simulink library "MOVH"  (R2016b)
settings: Solver=ode45  StartTime=0.0  StopTime=10.0  RelTol=1e-3  EnableMultiTasking=on
undefined symbols (not defined in the file): CAL_fullCircle_DEG, CAL_halfCircle_DEG, CAL_Kd, CAL_Ki, CAL_Kp, CAL_NO_ERROR, CAL_thetaGain, CONST_EnableDelay, CONST_NegOne, CONST_TWO_F32, CONST_ZERO_F32, ENU_BACKWARD, ENU_CCW, ENU_CW, ENU_FORWARD, ENU_MOVE_TURN_LEFT, ENU_MOVE_TURN_RIGHT, ENU_MOVE_U_TURN, ENU_MOVE_U_TURN_LEFT, ENU_MOVE_U_TURN_RIGHT, ENU_ROB_NONE, ENU_STOP
libraries: simulink_need_slupdate x2
settings Model: Creator=oelkawok  LastModifiedBy=oelkawok
settings DataIOCC: LimitDataPoints=on
settings OptimizationCC: LifeSpan=inf
settings DebuggingCC: AllowSymbolicDim=off  SFUnexpectedBacktrackingDiag=warning  SFNoUnconditionalDefaultTransitionDiag=warning  SFExecutionAtInitializationDiag=none
settings GRTTargetCC: TargetLangStandard=C89/C90 (ANSI)  GeneratePreprocessorConditionals=Disable all
settings ConfigComp: CovMetricSettings=dw  CovHtmlReporting=on  CovSaveCumulativeToWorkspaceVar=on  CovSaveSingleToWorkspaceVar=on  CovExternalEMLEnable=off

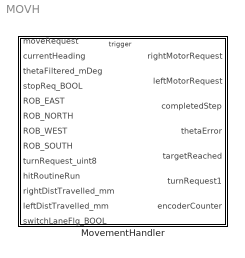
== system MOVH ==
  MovementHandler : Subsystem

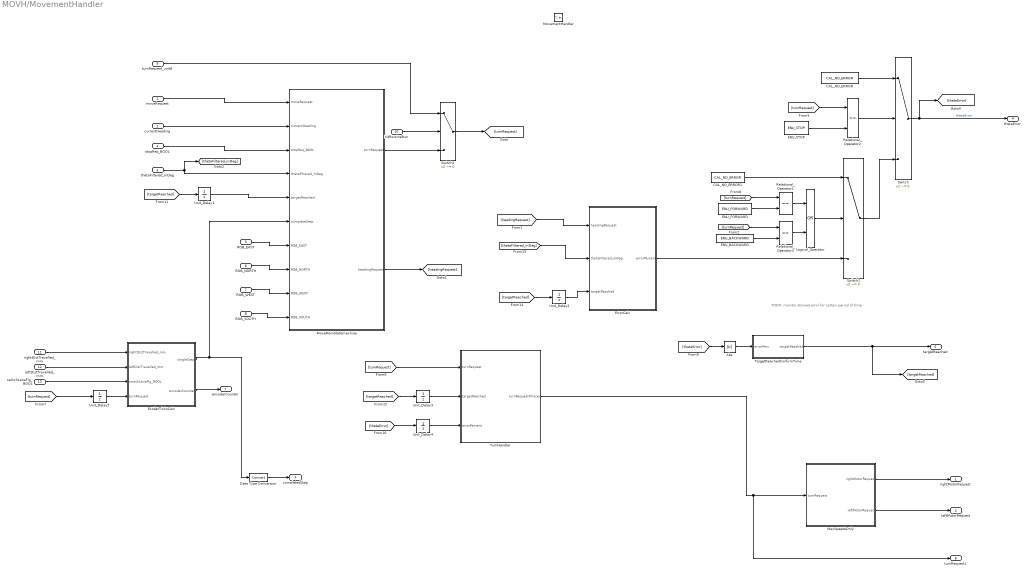
== system MOVH/MovementHandler ==
  note: TODO: monitor allowed error for certain period of time
  moveRequest : Inport
  currentHeading : Inport  Port=2
  thetaFiltered_mDeg : Inport  Port=3  PortDimensions=1
  stopReq_BOOL : Inport  Port=4
  ROB_EAST : Inport  Port=5  PortDimensions=1
  ROB_NORTH : Inport  Port=6  PortDimensions=1
  ROB_WEST : Inport  Port=7  PortDimensions=1
  ROB_SOUTH : Inport  Port=8  PortDimensions=1
  turnRequest_uint8 : Inport  Port=9
  hitRoutineRun : Inport  Port=10
  rightDistTravelled_mm : Inport  Port=11  PortDimensions=1
  leftDistTravelled_mm : Inport  Port=12  PortDimensions=1
  switchLaneFlg_BOOL : Inport  Port=13  PortDimensions=1
  MovementHandler : TriggerPort  TriggerType=function-call  VariantControl=Variant
      settings: AttributesFormatString=Mode: %<StatesWhenEnabling>
  Abs : Abs
  CAL_NO_ERROR : Constant  Value=CAL_NO_ERROR
  CAL_NO_ERROR1 : Constant  Value=CAL_NO_ERROR
  Data Type Conversion : DataTypeConversion
  ENU_BACKWARD : Constant  Value=ENU_BACKWARD
  ENU_FORWARD : Constant  Value=ENU_FORWARD
  ENU_STOP : Constant  Value=ENU_STOP
  EcoderTicksCalc : Subsystem
  ErrorCalc : Subsystem
  Logical_Operator : Logic  Operator=OR  AllPortsSameDT=off  OutDataTypeStr=boolean
  MaxSpeedsOnly : Subsystem
  MoveMainStatemachine : Subsystem
  Relational_Operator1 : RelationalOperator  Operator===  OutDataTypeStr=boolean  RndMeth=Nearest
  Relational_Operator2 : RelationalOperator  Operator===  OutDataTypeStr=boolean  RndMeth=Nearest
  Relational_Operator3 : RelationalOperator  Operator===  OutDataTypeStr=boolean  RndMeth=Nearest
  Switch : Switch  Criteria=u2 ~= 0
  Switch1 : Switch  Criteria=u2 ~= 0
  Switch2 : Switch  Criteria=u2 ~= 0
  TargetReachedConfirmTime : Subsystem
  TurnHandler : Subsystem
  Unit_Delay{1..4} (4 alike) : UnitDelay  InitialCondition=CAL_NO_ERROR  SampleTime=-1
      settings: AttributesFormatString=Init: %<InitialCondition>
  Unit_Delay5 : UnitDelay  InitialCondition=false  SampleTime=-1
      settings: AttributesFormatString=Init: %<InitialCondition>
  rightMotorRequest : Outport
      settings: AttributesFormatString=|
      | Mode: %<OutputWhenDisabled>
      | Init: %<InitialOutput>
  leftMotorRequest : Outport  Port=2
      settings: AttributesFormatString=|
      | Mode: %<OutputWhenDisabled>
      | Init: %<InitialOutput>
  completedStep : Outport  Port=3
      settings: AttributesFormatString=|
      | Mode: %<OutputWhenDisabled>
      | Init: %<InitialOutput>
  thetaError : Outport  Port=4  OutputWhenDisabled=reset  InitialOutput=0
      settings: AttributesFormatString=|
      | Mode: %<OutputWhenDisabled>
      | Init: %<InitialOutput>
  targetReached : Outport  Port=5  OutputWhenDisabled=reset  InitialOutput=0
      settings: AttributesFormatString=|
      | Mode: %<OutputWhenDisabled>
      | Init: %<InitialOutput>
  turnRequest1 : Outport  Port=6
      settings: AttributesFormatString=|
      | Mode: %<OutputWhenDisabled>
      | Init: %<InitialOutput>
  encoderCounter : Outport  Port=7
      settings: AttributesFormatString=|
      | Mode: %<OutputWhenDisabled>
      | Init: %<InitialOutput>
  wires:
  Logical_Operator/1 -> Switch1/2
  Abs/1 -> TargetReachedConfirmTime/1(errorPerc)
  TargetReachedConfirmTime/1(targetReached) -> targetReached/1, [targetReached]
  Data Type Conversion/1 -> completedStep/1
  Unit_Delay1/1 -> MoveMainStatemachine/5(targetReached)
  [targetReached] -> Unit_Delay1/1
  [thetaFiltered_mDeg] -> ErrorCalc/2(thetaFiltered_mDeg)
  thetaFiltered_mDeg/1 -> [thetaFiltered_mDeg], MoveMainStatemachine/4(thetaFiltered_mDeg)
  currentHeading/1 -> MoveMainStatemachine/2(currentHeading)
  MoveMainStatemachine/2(headingRequest) -> [headingRequest]
  MoveMainStatemachine/1(turnRequest) -> Switch2/3
  stopReq_BOOL/1 -> MoveMainStatemachine/3(stopReq_BOOL)
  moveRequest/1 -> MoveMainStatemachine/1(moveRequest)
  MaxSpeedsOnly/1(rightMotorRequest) -> rightMotorRequest/1
  MaxSpeedsOnly/2(leftMotorRequest) -> leftMotorRequest/1
  [turnRequest] -> TurnHandler/1(turnRequest)
  [headingRequest] -> ErrorCalc/1(headingRequest)
  ENU_STOP/1 -> Relational_Operator2/2
  [turnRequest] -> Relational_Operator2/1
  Relational_Operator2/1 -> Switch/2
  CAL_NO_ERROR/1 -> Switch/1
  Switch1/1 -> Switch/3
  [turnRequest] -> Relational_Operator1/1
  ErrorCalc/1(errorPercent) -> Switch1/3
  Switch/1 -> [thetaError], thetaError/1  "thetaError"
  [thetaError] -> Abs/1
  [targetReached] -> Unit_Delay2/1
  Unit_Delay2/1 -> ErrorCalc/3(targetReached)
  [targetReached] -> Unit_Delay3/1
  Unit_Delay3/1 -> TurnHandler/2(targetReached)
  Unit_Delay4/1 -> TurnHandler/3(errorPercent)
  [thetaError] -> Unit_Delay4/1
  TurnHandler/1(turnRequestFiltered) -> MaxSpeedsOnly/1(turnRequest), turnRequest1/1
  CAL_NO_ERROR1/1 -> Switch1/1
  EcoderTicksCalc/1(singleStep) -> Data Type Conversion/1, MoveMainStatemachine/6(completeStep)
  ROB_EAST/1 -> MoveMainStatemachine/7(ROB_EAST)
  ROB_NORTH/1 -> MoveMainStatemachine/8(ROB_NORTH)
  ROB_WEST/1 -> MoveMainStatemachine/9(ROB_WEST)
  ROB_SOUTH/1 -> MoveMainStatemachine/10(ROB_SOUTH)
  turnRequest_uint8/1 -> Switch2/1
  Switch2/1 -> [turnRequest]
  hitRoutineRun/1 -> Switch2/2
  EcoderTicksCalc/2(encoderCounter) -> encoderCounter/1
  [turnRequest] -> Unit_Delay5/1
  ENU_FORWARD/1 -> Relational_Operator1/2
  ENU_BACKWARD/1 -> Relational_Operator3/2
  [turnRequest] -> Relational_Operator3/1
  Relational_Operator1/1 -> Logical_Operator/1
  Relational_Operator3/1 -> Logical_Operator/2
  Unit_Delay5/1 -> EcoderTicksCalc/4(turnRequest)
  rightDistTravelled_mm/1 -> EcoderTicksCalc/1(rightDistTravelled_mm)
  leftDistTravelled_mm/1 -> EcoderTicksCalc/2(leftDistTravelled_mm)
  switchLaneFlg_BOOL/1 -> EcoderTicksCalc/3(switchLaneFlg_BOOL)

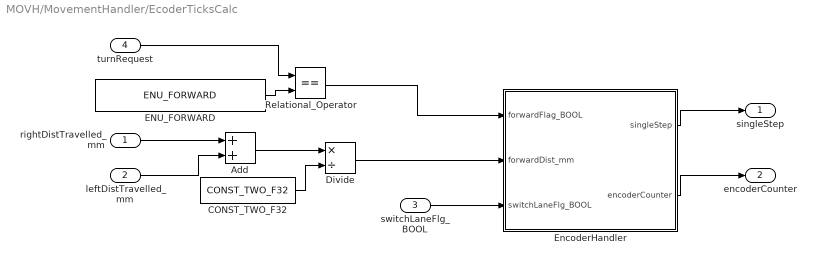
== system MOVH/MovementHandler/EcoderTicksCalc ==
  rightDistTravelled_mm : Inport  PortDimensions=1
  leftDistTravelled_mm : Inport  Port=2  PortDimensions=1
  switchLaneFlg_BOOL : Inport  Port=3  PortDimensions=1
  turnRequest : Inport  Port=4  PortDimensions=1
  Add : Sum
  CONST_TWO_F32 : Constant  Value=CONST_TWO_F32
  Divide : Product  Inputs=*/
  ENU_FORWARD : Constant  Value=ENU_FORWARD
  EncoderHandler : Subsystem
  Relational_Operator : RelationalOperator  Operator===  OutDataTypeStr=boolean  RndMeth=Simplest
  singleStep : Outport
  encoderCounter : Outport  Port=2
  wires:
  EncoderHandler/1(singleStep) -> singleStep/1
  EncoderHandler/2(encoderCounter) -> encoderCounter/1
  turnRequest/1 -> Relational_Operator/1
  rightDistTravelled_mm/1 -> Add/1
  leftDistTravelled_mm/1 -> Add/2
  Add/1 -> Divide/1
  CONST_TWO_F32/1 -> Divide/2
  ENU_FORWARD/1 -> Relational_Operator/2
  Divide/1 -> EncoderHandler/2(forwardDist_mm)
  switchLaneFlg_BOOL/1 -> EncoderHandler/3(switchLaneFlg_BOOL)
  Relational_Operator/1 -> EncoderHandler/1(forwardFlag_BOOL)

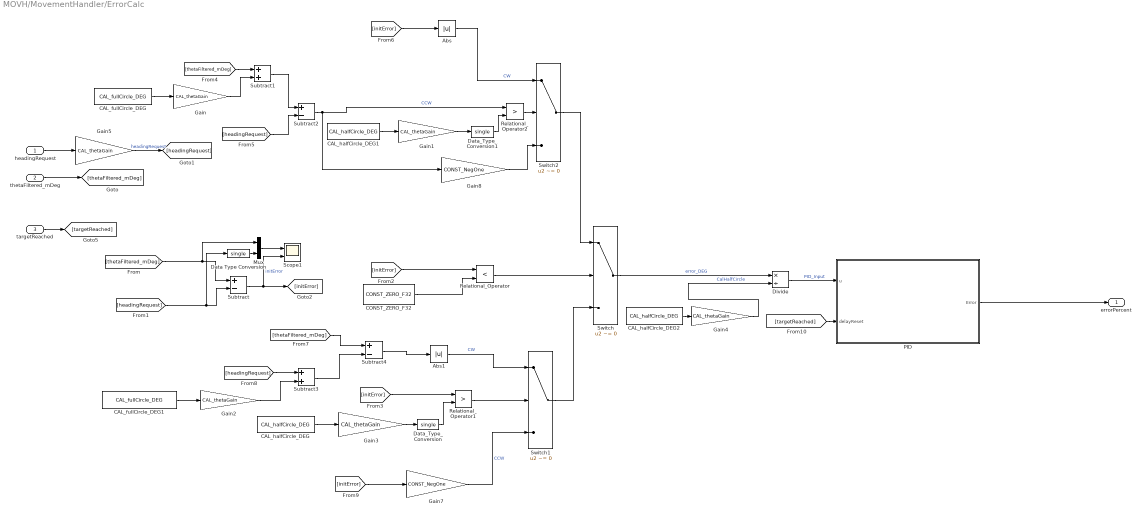
== system MOVH/MovementHandler/ErrorCalc ==
  headingRequest : Inport
  thetaFiltered_mDeg : Inport  Port=2
  targetReached : Inport  Port=3
  Abs : Abs
  Abs1 : Abs
  CAL_fullCircle_DEG : Constant  Value=CAL_fullCircle_DEG
  CAL_fullCircle_DEG1 : Constant  Value=CAL_fullCircle_DEG
  CAL_halfCircle_DEG : Constant  Value=CAL_halfCircle_DEG
  CAL_halfCircle_DEG1 : Constant  Value=CAL_halfCircle_DEG
  CAL_halfCircle_DEG2 : Constant  Value=CAL_halfCircle_DEG
  CONST_ZERO_F32 : Constant  Value=CONST_ZERO_F32
  Data Type Conversion : DataTypeConversion  OutDataTypeStr=single
  Data_Type_Conversion : DataTypeConversion  OutDataTypeStr=single
  Data_Type_Conversion1 : DataTypeConversion  OutDataTypeStr=single
  Divide : Product  Inputs=*/
  Gain : Gain  Gain=CAL_thetaGain  OutDataTypeStr=int32
  Gain1 : Gain  Gain=CAL_thetaGain  OutDataTypeStr=int16
  Gain2 : Gain  Gain=CAL_thetaGain  OutDataTypeStr=int32
  Gain3 : Gain  Gain=CAL_thetaGain  OutDataTypeStr=Inherit: Inherit via back propagation
  Gain4 : Gain  Gain=CAL_thetaGain  OutDataTypeStr=int16
  Gain5 : Gain  Gain=CAL_thetaGain  OutDataTypeStr=int32
  Gain7 : Gain  Gain=CONST_NegOne
  Gain8 : Gain  Gain=CONST_NegOne
  Mux : Mux  Inputs=2
  PID : Subsystem
  Relational_Operator : RelationalOperator  Operator=<  OutDataTypeStr=boolean  RndMeth=Nearest
  Relational_Operator1 : RelationalOperator  Operator=>  OutDataTypeStr=boolean  RndMeth=Nearest
  Relational_Operator2 : RelationalOperator  Operator=>  OutDataTypeStr=boolean  RndMeth=Nearest
  Scope1 : Scope  NumInputPorts=2
  Subtract : Sum  Inputs=+-
  Subtract1 : Sum
  Subtract2 : Sum  Inputs=+-
  Subtract3 : Sum  OutDataTypeStr=int32
  Subtract4 : Sum  Inputs=+-
  Switch : Switch  Criteria=u2 ~= 0
  Switch1 : Switch  Criteria=u2 ~= 0
  Switch2 : Switch  Criteria=u2 ~= 0
  errorPercent : Outport  OutputWhenDisabled=reset  InitialOutput=0
  wires:
  Data Type Conversion/1 -> Mux/2
  Mux/1 -> Scope1/1
  CAL_halfCircle_DEG2/1 -> Gain4/1
  Switch/1 -> Divide/1  "error_DEG"
  [initError] -> Gain7/1
  Abs1/1 -> Switch1/1  "CW"
  Subtract4/1 -> Abs1/1
  Subtract3/1 -> Subtract4/2
  [thetaFiltered_mDeg] -> Subtract4/1
  [headingRequest] -> Subtract3/1
  CAL_fullCircle_DEG1/1 -> Gain2/1
  Abs/1 -> Switch2/1  "CW"
  [initError] -> Abs/1
  Switch2/1 -> Switch/1
  Relational_Operator2/1 -> Switch2/2
  Subtract2/1 -> Relational_Operator2/1, Gain8/1  "CCW"
  CAL_halfCircle_DEG1/1 -> Gain1/1
  [headingRequest] -> Subtract2/2
  Subtract1/1 -> Subtract2/1
  CAL_fullCircle_DEG/1 -> Gain/1
  [thetaFiltered_mDeg] -> Subtract1/1
  [initError] -> Relational_Operator1/1
  [initError] -> Relational_Operator/1
  Subtract/1 -> [initError], Scope1/2  "initError"
  [thetaFiltered_mDeg] -> Subtract/1, Mux/1
  [headingRequest] -> Subtract/2, Data Type Conversion/1
  thetaFiltered_mDeg/1 -> [thetaFiltered_mDeg]
  headingRequest/1 -> Gain5/1
  Switch1/1 -> Switch/3
  CAL_halfCircle_DEG/1 -> Gain3/1
  Relational_Operator1/1 -> Switch1/2
  Relational_Operator/1 -> Switch/2
  CONST_ZERO_F32/1 -> Relational_Operator/2
  Gain/1 -> Subtract1/2
  Gain1/1 -> Data_Type_Conversion1/1
  Gain2/1 -> Subtract3/2
  Gain3/1 -> Data_Type_Conversion/1
  Gain5/1 -> [headingRequest]  "headingRequest"
  targetReached/1 -> [targetReached]
  Gain7/1 -> Switch1/3  "CCW"
  Gain8/1 -> Switch2/3
  PID/1(Error) -> errorPercent/1
  Divide/1 -> PID/1(u)  "PID_Input"
  [targetReached] -> PID/2(delayReset)
  Gain4/1 -> Divide/2  "CalHalfCircle"
  Data_Type_Conversion/1 -> Relational_Operator1/2
  Data_Type_Conversion1/1 -> Relational_Operator2/2

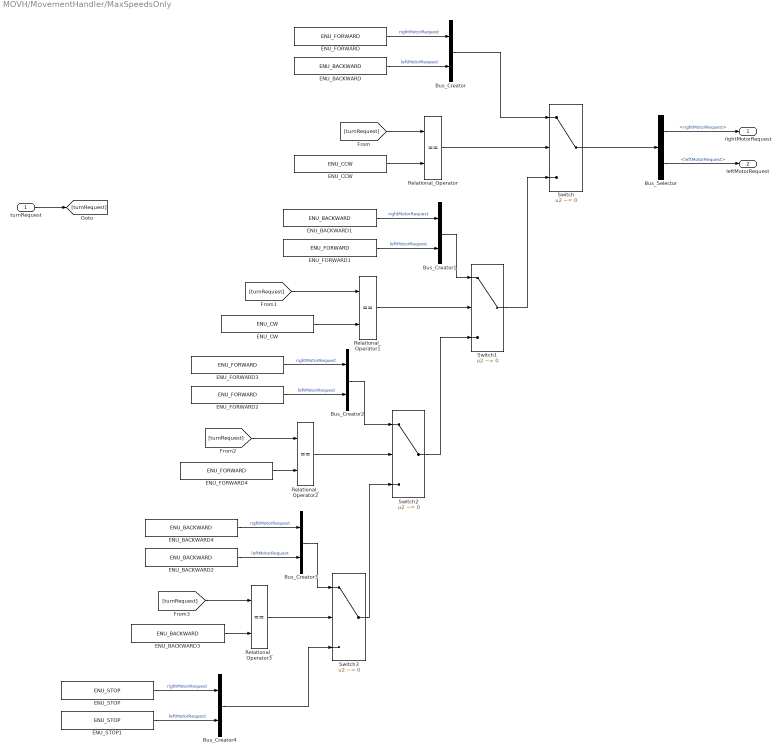
== system MOVH/MovementHandler/MaxSpeedsOnly ==
  turnRequest : Inport
  Bus_Creator{,1..4} (5 alike) : BusCreator  Inputs=2
  Bus_Selector : BusSelector  OutputSignals=rightMotorRequest,leftMotorRequest
  ENU_BACKWARD{,1..4} (5 alike) : Constant  Value=ENU_BACKWARD
  ENU_CCW : Constant  Value=ENU_CCW
  ENU_CW : Constant  Value=ENU_CW
  ENU_FORWARD{,1..4} (5 alike) : Constant  Value=ENU_FORWARD
  ENU_STOP : Constant  Value=ENU_STOP
  ENU_STOP1 : Constant  Value=ENU_STOP
  Relational_Operator{,1..3} (4 alike) : RelationalOperator  Operator===  OutDataTypeStr=boolean  RndMeth=Nearest
  Switch{,1..3} (4 alike) : Switch  Criteria=u2 ~= 0
  rightMotorRequest : Outport
  leftMotorRequest : Outport  Port=2
  wires:
  ENU_FORWARD/1 -> Bus_Creator/1  "rightMotorRequest"
  ENU_CCW/1 -> Relational_Operator/2
  Relational_Operator/1 -> Switch/2
  [turnRequest] -> Relational_Operator/1
  Switch/1 -> Bus_Selector/1
  ENU_BACKWARD/1 -> Bus_Creator/2  "leftMotorRequest"
  Bus_Creator/1 -> Switch/1
  [turnRequest] -> Relational_Operator1/1
  Bus_Selector/1 -> rightMotorRequest/1  "<rightMotorRequest>"
  ENU_FORWARD1/1 -> Bus_Creator1/2  "leftMotorRequest"
  Bus_Selector/2 -> leftMotorRequest/1  "<leftMotorRequest>"
  Switch1/1 -> Switch/3
  [turnRequest] -> Relational_Operator3/1
  ENU_BACKWARD1/1 -> Bus_Creator1/1  "rightMotorRequest"
  Bus_Creator1/1 -> Switch1/1
  ENU_CW/1 -> Relational_Operator1/2
  ENU_FORWARD3/1 -> Bus_Creator2/1  "rightMotorRequest"
  Relational_Operator1/1 -> Switch1/2
  Relational_Operator3/1 -> Switch3/2
  [turnRequest] -> Relational_Operator2/1
  ENU_FORWARD4/1 -> Relational_Operator2/2
  Switch2/1 -> Switch1/3
  Relational_Operator2/1 -> Switch2/2
  ENU_BACKWARD4/1 -> Bus_Creator3/1  "rightMotorRequest"
  ENU_BACKWARD2/1 -> Bus_Creator3/2  "leftMotorRequest"
  ENU_BACKWARD3/1 -> Relational_Operator3/2
  Bus_Creator2/1 -> Switch2/1
  Bus_Creator4/1 -> Switch3/3
  Switch3/1 -> Switch2/3
  ENU_STOP1/1 -> Bus_Creator4/2  "leftMotorRequest"
  Bus_Creator3/1 -> Switch3/1
  ENU_FORWARD2/1 -> Bus_Creator2/2  "leftMotorRequest"
  ENU_STOP/1 -> Bus_Creator4/1  "rightMotorRequest"
  turnRequest/1 -> [turnRequest]

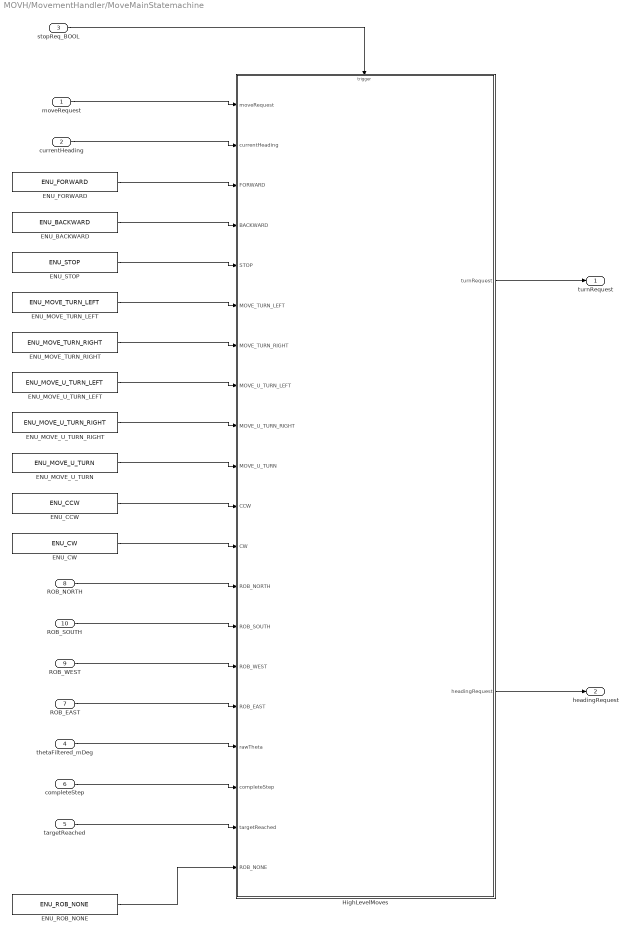
== system MOVH/MovementHandler/MoveMainStatemachine ==
  moveRequest : Inport
  currentHeading : Inport  Port=2
  stopReq_BOOL : Inport  Port=3
  thetaFiltered_mDeg : Inport  Port=4  PortDimensions=1
  targetReached : Inport  Port=5  PortDimensions=1
  completeStep : Inport  Port=6  PortDimensions=1
  ROB_EAST : Inport  Port=7  PortDimensions=1
  ROB_NORTH : Inport  Port=8  PortDimensions=1
  ROB_WEST : Inport  Port=9  PortDimensions=1
  ROB_SOUTH : Inport  Port=10  PortDimensions=1
  ENU_BACKWARD : Constant  Value=ENU_BACKWARD
  ENU_CCW : Constant  Value=ENU_CCW
  ENU_CW : Constant  Value=ENU_CW
  ENU_FORWARD : Constant  Value=ENU_FORWARD
  ENU_MOVE_TURN_LEFT : Constant  Value=ENU_MOVE_TURN_LEFT
  ENU_MOVE_TURN_RIGHT : Constant  Value=ENU_MOVE_TURN_RIGHT
  ENU_MOVE_U_TURN : Constant  Value=ENU_MOVE_U_TURN
  ENU_MOVE_U_TURN_LEFT : Constant  Value=ENU_MOVE_U_TURN_LEFT
  ENU_MOVE_U_TURN_RIGHT : Constant  Value=ENU_MOVE_U_TURN_RIGHT
  ENU_ROB_NONE : Constant  Value=ENU_ROB_NONE
  ENU_STOP : Constant  Value=ENU_STOP
  HighLevelMoves : Stateflow chart  TreatAsAtomicUnit=on
  turnRequest : Outport
  headingRequest : Outport  Port=2
  wires:
  targetReached/1 -> HighLevelMoves/19(targetReached)
  thetaFiltered_mDeg/1 -> HighLevelMoves/17(rawTheta)
  completeStep/1 -> HighLevelMoves/18(completeStep)
  ENU_CW/1 -> HighLevelMoves/12(CW)
  ENU_MOVE_U_TURN_RIGHT/1 -> HighLevelMoves/9(MOVE_U_TURN_RIGHT)
  ENU_MOVE_U_TURN_LEFT/1 -> HighLevelMoves/8(MOVE_U_TURN_LEFT)
  ENU_MOVE_TURN_LEFT/1 -> HighLevelMoves/6(MOVE_TURN_LEFT)
  ENU_BACKWARD/1 -> HighLevelMoves/4(BACKWARD)
  ENU_FORWARD/1 -> HighLevelMoves/3(FORWARD)
  ENU_STOP/1 -> HighLevelMoves/5(STOP)
  ENU_MOVE_TURN_RIGHT/1 -> HighLevelMoves/7(MOVE_TURN_RIGHT)
  currentHeading/1 -> HighLevelMoves/2(currentHeading)
  moveRequest/1 -> HighLevelMoves/1(moveRequest)
  HighLevelMoves/2(headingRequest) -> headingRequest/1
  ROB_WEST/1 -> HighLevelMoves/15(ROB_WEST)
  ROB_SOUTH/1 -> HighLevelMoves/14(ROB_SOUTH)
  ROB_NORTH/1 -> HighLevelMoves/13(ROB_NORTH)
  ENU_CCW/1 -> HighLevelMoves/11(CCW)
  ROB_EAST/1 -> HighLevelMoves/16(ROB_EAST)
  ENU_MOVE_U_TURN/1 -> HighLevelMoves/10(MOVE_U_TURN)
  ENU_ROB_NONE/1 -> HighLevelMoves/20(ROB_NONE)
  HighLevelMoves/1(turnRequest) -> turnRequest/1
  stopReq_BOOL/1 -> HighLevelMoves/Trigger

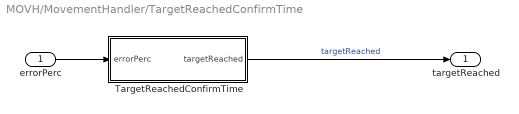
== system MOVH/MovementHandler/TargetReachedConfirmTime ==
  errorPerc : Inport
  TargetReachedConfirmTime : Stateflow chart  TreatAsAtomicUnit=on
  targetReached : Outport
  wires:
  errorPerc/1 -> TargetReachedConfirmTime/1(errorPerc)
  TargetReachedConfirmTime/1(targetReached) -> targetReached/1  "targetReached"

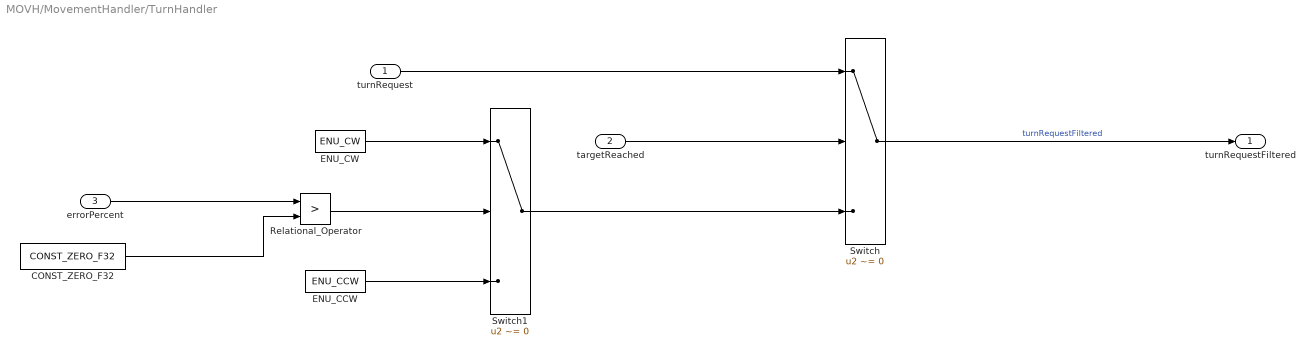
== system MOVH/MovementHandler/TurnHandler ==
  turnRequest : Inport
  targetReached : Inport  Port=2
  errorPercent : Inport  Port=3
  CONST_ZERO_F32 : Constant  Value=CONST_ZERO_F32
  ENU_CCW : Constant  Value=ENU_CCW
  ENU_CW : Constant  Value=ENU_CW
  Relational_Operator : RelationalOperator  Operator=>  OutDataTypeStr=boolean  RndMeth=Nearest
  Switch : Switch  Criteria=u2 ~= 0
  Switch1 : Switch  Criteria=u2 ~= 0
  turnRequestFiltered : Outport
  wires:
  targetReached/1 -> Switch/2
  Switch1/1 -> Switch/3
  Relational_Operator/1 -> Switch1/2
  errorPercent/1 -> Relational_Operator/1
  CONST_ZERO_F32/1 -> Relational_Operator/2
  turnRequest/1 -> Switch/1
  Switch/1 -> turnRequestFiltered/1  "turnRequestFiltered"
  ENU_CCW/1 -> Switch1/3
  ENU_CW/1 -> Switch1/1

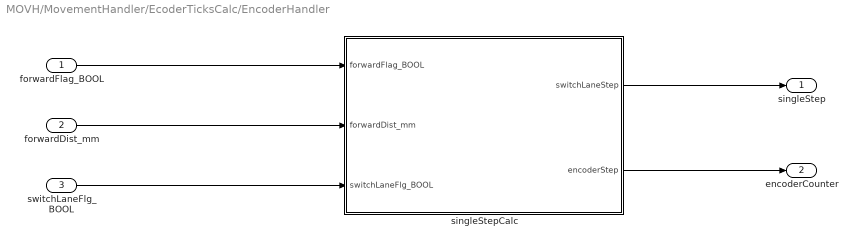
== system MOVH/MovementHandler/EcoderTicksCalc/EncoderHandler ==
  forwardFlag_BOOL : Inport  PortDimensions=1
  forwardDist_mm : Inport  Port=2
  switchLaneFlg_BOOL : Inport  Port=3  PortDimensions=1
  singleStepCalc : Stateflow chart  TreatAsAtomicUnit=on
  singleStep : Outport  OutputWhenDisabled=reset  InitialOutput=0
  encoderCounter : Outport  Port=2  OutputWhenDisabled=reset  InitialOutput=0
  wires:
  singleStepCalc/1(switchLaneStep) -> singleStep/1
  forwardDist_mm/1 -> singleStepCalc/2(forwardDist_mm)
  forwardFlag_BOOL/1 -> singleStepCalc/1(forwardFlag_BOOL)
  switchLaneFlg_BOOL/1 -> singleStepCalc/3(switchLaneFlg_BOOL)
  singleStepCalc/2(encoderStep) -> encoderCounter/1

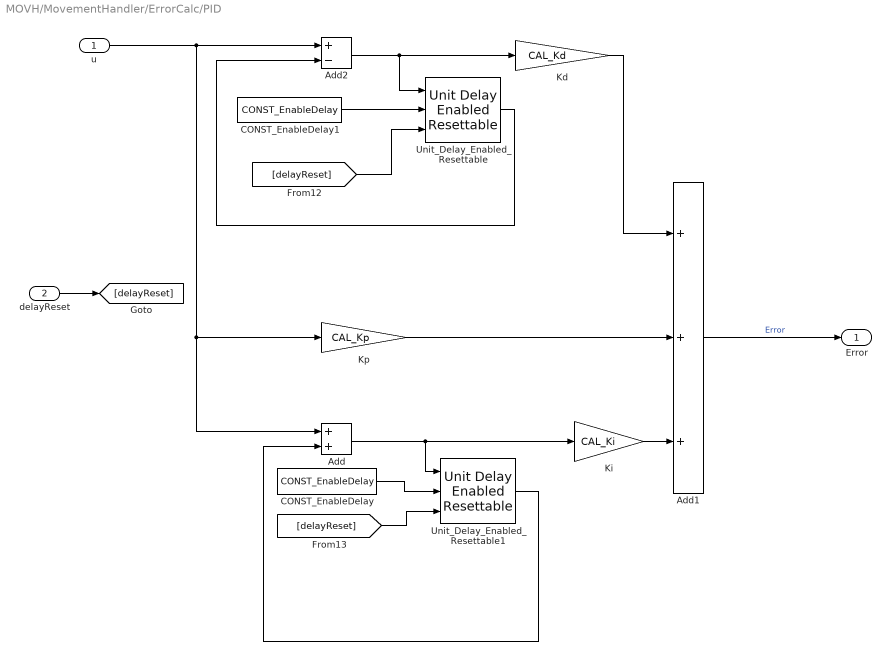
== system MOVH/MovementHandler/ErrorCalc/PID ==
  u : Inport
  delayReset : Inport  Port=2
  Add : Sum
  Add1 : Sum  Inputs=+++  OutDataTypeStr=single
  Add2 : Sum  Inputs=+-
  CONST_EnableDelay : Constant  Value=CONST_EnableDelay
  CONST_EnableDelay1 : Constant  Value=CONST_EnableDelay
  Kd : Gain  Gain=CAL_Kd
  Ki : Gain  Gain=CAL_Ki
  Kp : Gain  Gain=CAL_Kp
  Unit_Delay_Enabled_Resettable : simulink_need_slupdate/Unit Delay Enabled Resettable  vinit=0.0  tsamp=-1
  Unit_Delay_Enabled_Resettable1 : simulink_need_slupdate/Unit Delay Enabled Resettable  vinit=0.0  tsamp=-1
  Error : Outport
  wires:
  u/1 -> Kp/1, Add/1, Add2/1
  Add/1 -> Unit_Delay_Enabled_Resettable1/1, Ki/1
  Unit_Delay_Enabled_Resettable1/1 -> Add/2
  Ki/1 -> Add1/3
  Add2/1 -> Unit_Delay_Enabled_Resettable/1, Kd/1
  Unit_Delay_Enabled_Resettable/1 -> Add2/2
  Kd/1 -> Add1/1
  Kp/1 -> Add1/2
  Add1/1 -> Error/1  "Error"
  CONST_EnableDelay1/1 -> Unit_Delay_Enabled_Resettable/2
  [delayReset] -> Unit_Delay_Enabled_Resettable/3
  CONST_EnableDelay/1 -> Unit_Delay_Enabled_Resettable1/2
  [delayReset] -> Unit_Delay_Enabled_Resettable1/3
  delayReset/1 -> [delayReset]

== stateflow chart MOVH/MovementHandler/TargetReachedConfirmTime/TargetReachedConfirmTime ==
  settings: description=time needed to confirm steady state for the PID
  (default) -> (junction 1)
  (junction 1) -> (junction 3) [order 1] : [errorPerc <= CAL_ALLOWED_ERROR_VALUE]
  (junction 1) -> (junction 12) [order 2] : {
      | counter = 0;
      | targetReached = false;
      | }
  (junction 3) -> (junction 5) : {
      | counter++;
      | }
  (junction 5) -> (junction 10) [order 1] : [counter > CONST_TARGET_REACHED_TIMER]
  (junction 5) -> (junction 20) [order 2]
  (junction 10) -> (junction 11) : {
      | counter = 0;
      | targetReached = true;
      | }
  (junction 20) -> (junction 12)
  (junction 11) -> (junction 20)
  data: errorPerc input; counter local uint8; CAL_ALLOWED_ERROR_VALUE constant single =CAL_ALLOWED_ERROR_VALUE; targetReached output boolean; CONST_TARGET_REACHED_TIMER constant single =CONST_TARGET_REACHED_TIMER

== stateflow chart MOVH/MovementHandler/EcoderTicksCalc/EncoderHandler/singleStepCalc ==
  settings: description=calculating single step the robot moves in straight line mainlt forward state. to it update the sensor view and also gives change lane step
  state ForwardStep
    en:
    encoderStep = true;
  state waitingSwitchLane
  state initiateDist
    en:
    tempDistance_mm = forwardDist_mm;
    encoderStep = false;
  state SwitchLaneStep
    en:
    switchLaneStep = true;
  ForwardStep -> waitingSwitchLane
  initiateDist -> ForwardStep [order 2] : [!switchLaneFlg_BOOL && (forwardDist_mm - tempDistance_mm) >= (CAL_BLOCK_SIZE_mm * CONST_SNSR_VIEW_PERC)]
  (default) -> waitingSwitchLane
  initiateDist -> waitingSwitchLane [order 3] : [!forwardFlag_BOOL]
  waitingSwitchLane -> initiateDist : [forwardFlag_BOOL]
  initiateDist -> SwitchLaneStep [order 1] : [switchLaneFlg_BOOL && (forwardDist_mm - tempDistance_mm) >= CAL_BLOCK_SIZE_mm]
  SwitchLaneStep -> waitingSwitchLane : [!switchLaneFlg_BOOL]
      | /switchLaneStep = false;
  data: forwardFlag_BOOL input; switchLaneStep output boolean; forwardDist_mm input; CAL_BLOCK_SIZE_mm constant uint8 =CAL_BLOCK_SIZE_mm; encoderStep output uint8; tempDistance_mm local single; switchLaneFlg_BOOL input; CONST_SNSR_VIEW_PERC constant single =CONST_SNSR_VIEW_PERC

== stateflow chart MOVH/MovementHandler/MoveMainStatemachine/HighLevelMoves ==
  settings: description=movement state machine handles all the movement in slightly higher level. turn left , right, stop, forward, backward and also combinations like u-turn left u-turn right
  state init
    en:
    stableCounter = 0;
    turnRequest = STOP;
    headingRequest = ROB_NONE;
    currentMove = STOP;
    du:
    stableCounter++;
  state Stop
  state forward
    state fixingHeading
    state Idle
    (junction 252) -> fixingHeading [order 1] : [(rawTheta < ROB_SOUTH*CAL_thetaGain)...
        | || (rawTheta > ROB_NORTH*CAL_thetaGain)]
        | /turnRequest = CCW;
    (default) -> Idle
    (junction 252) -> fixingHeading [order 2] : /turnRequest = CW;
    (junction 250) -> (junction 252) [order 1] : [headingRequest == ROB_NORTH]
    (junction 253) -> fixingHeading [order 1] : [(rawTheta < ROB_SOUTH*CAL_thetaGain)...
        | || (rawTheta > ROB_NORTH*CAL_thetaGain)]
        | /turnRequest = CW;
    (junction 250) -> (junction 253) [order 2] : [headingRequest == ROB_SOUTH]
    (junction 253) -> fixingHeading [order 2] : /turnRequest = CCW;
    Idle -> (junction 270)
    (junction 270) -> (junction 250) [order 1] : [!((rawTheta >= (headingRequest*CAL_thetaGain) - CAL_forwardThetaThd)...
        | && (rawTheta <= (headingRequest*CAL_thetaGain) + CAL_forwardThetaThd))]
    (junction 250) -> (junction 254) [order 3] : [headingRequest == ROB_EAST]
    (junction 270) -> Idle [order 2] : [(rawTheta >= (headingRequest*CAL_thetaGain) - CAL_forwardThetaThd)...
        | && (rawTheta <= (headingRequest*CAL_thetaGain) + CAL_forwardThetaThd)]
        | /turnRequest = FORWARD;
    (junction 250) -> (junction 255) [order 4] : [headingRequest == ROB_WEST]
    (junction 254) -> fixingHeading [order 1] : [rawTheta > ROB_WEST*CAL_thetaGain]
        | /turnRequest = CW;
    (junction 254) -> fixingHeading [order 2] : /turnRequest = CCW;
    (junction 255) -> fixingHeading [order 1] : [rawTheta > ROB_WEST*CAL_thetaGain]
        | /turnRequest = CCW;
    fixingHeading -> Idle
    (junction 255) -> fixingHeading [order 2] : /turnRequest = CW;
  state TurnLeft
    state finish
      entry:
      turnActive = false;
    state start
      entry:
      turnRequest = CCW;
      turnActive = true;
    state turning
    (default) -> TurnLeft.start
    TurnLeft.start -> TurnLeft.turning [order 1] : [currentHeading == ROB_NORTH]
        | /headingRequest = ROB_WEST;
    TurnLeft.start -> TurnLeft.turning [order 3] : [currentHeading == ROB_SOUTH]
        | /headingRequest = ROB_EAST;
    TurnLeft.turning -> TurnLeft.finish : [(currentHeading == headingRequest)...
        | && (targetReached == true)]
    TurnLeft.start -> TurnLeft.turning [order 4] : [currentHeading == ROB_WEST]
        | /headingRequest = ROB_SOUTH;
    TurnLeft.start -> TurnLeft.turning [order 2] : [currentHeading == ROB_EAST]
        | /headingRequest = ROB_NORTH;
  state backward
  state UturnLeft
    entry:
    uTurnCounter = 0;
    state finish
      entry:
      turnActive = false;
    state TurnLeft
      state finish
        entry:
        uTurnCounter := uTurnCounter + 1;
      state start
        entry:
        turnRequest = CCW;
        turnActive = true;
      state turning
      (default) -> UturnLeft.TurnLeft.start
      UturnLeft.TurnLeft.start -> UturnLeft.TurnLeft.turning [order 1] : [currentHeading == ROB_NORTH]
          | /headingRequest = ROB_WEST;
      UturnLeft.TurnLeft.start -> UturnLeft.TurnLeft.turning [order 3] : [currentHeading == ROB_SOUTH]
          | /headingRequest = ROB_EAST;
      UturnLeft.TurnLeft.turning -> UturnLeft.TurnLeft.finish : [(currentHeading == headingRequest)...
          | && (targetReached == true)]
      UturnLeft.TurnLeft.start -> UturnLeft.TurnLeft.turning [order 4] : [currentHeading == ROB_WEST]
          | /headingRequest = ROB_SOUTH;
      UturnLeft.TurnLeft.start -> UturnLeft.TurnLeft.turning [order 2] : [currentHeading == ROB_EAST]
          | /headingRequest = ROB_NORTH;
    state forwardStep
      entry:
      //counter = 0;
      turnRequest = FORWARD;
      currentMove = FORWARD;
      du:
      //counter++;
    (default) -> UturnLeft.TurnLeft
    UturnLeft.TurnLeft -> UturnLeft.finish [order 2] : [uTurnCounter == CONST_UTURN_CNT_THD]
    UturnLeft.TurnLeft -> UturnLeft.forwardStep [order 1] : [(uTurnCounter == 1)...
        | && hasChanged(uTurnCounter)]
    UturnLeft.forwardStep -> UturnLeft.TurnLeft [order 2] : stopEvent
        | /currentMove = MOVE_U_TURN_LEFT;
    UturnLeft.forwardStep -> UturnLeft.TurnLeft [order 1] : [(hasChanged(completeStep))...
        | && (completeStep == true)]
        | /currentMove = MOVE_U_TURN_LEFT;
  state Uturn
    entry:
    uTurnCounter = 0;
    state finish
      entry:
      turnActive = false;
    state TurnRight
      state finish
        entry:
        uTurnCounter := uTurnCounter + 1;
        turnActive = false;
      state turning
      state start
        entry:
        turnRequest = CW;
        turnActive = true;
      (default) -> Uturn.TurnRight.start
      Uturn.TurnRight.start -> Uturn.TurnRight.turning [order 2] : [currentHeading == ROB_NORTH]
          | //headingRequest = ROB_EAST;
          | /headingRequest = ROB_SOUTH;
      Uturn.TurnRight.start -> Uturn.TurnRight.turning [order 4] : [currentHeading == ROB_SOUTH]
          | //headingRequest = ROB_WEST;
          | /headingRequest = ROB_NORTH;
      Uturn.TurnRight.turning -> Uturn.TurnRight.finish : [(currentHeading == headingRequest)...
          | && (targetReached == true)]
      Uturn.TurnRight.start -> Uturn.TurnRight.turning [order 3] : [currentHeading == ROB_WEST]
          | /headingRequest = ROB_NORTH;
      Uturn.TurnRight.start -> Uturn.TurnRight.turning [order 1] : [currentHeading == ROB_EAST]
          | /headingRequest = ROB_SOUTH;
    (default) -> Uturn.TurnRight
    Uturn.TurnRight -> Uturn.finish : [uTurnCounter == CONST_UTURN_CNT_THD]
  state TurnRight
    state turning
    state finish
      entry:
      turnActive = false;
    state start
      entry:
      turnRequest = CW;
      turnActive = true;
    (default) -> TurnRight.start
    TurnRight.start -> TurnRight.turning [order 2] : [currentHeading == ROB_NORTH]
        | /headingRequest = ROB_EAST;
    TurnRight.start -> TurnRight.turning [order 4] : [currentHeading == ROB_SOUTH]
        | /headingRequest = ROB_WEST;
    TurnRight.turning -> TurnRight.finish : [(currentHeading == headingRequest)...
        | && (targetReached == true)]
    TurnRight.start -> TurnRight.turning [order 3] : [currentHeading == ROB_WEST]
        | /headingRequest = ROB_NORTH;
    TurnRight.start -> TurnRight.turning [order 1] : [currentHeading == ROB_EAST]
        | /headingRequest = ROB_SOUTH;
  state UturnRight
    entry:
    uTurnCounter = 0;
    state finish
      entry:
      turnActive = false;
    state TurnRight
      state start
        entry:
        turnRequest = CW;
        turnActive = true;
      state finish
        entry:
        uTurnCounter := uTurnCounter + 1;
      state turning
      (default) -> UturnRight.TurnRight.start
      UturnRight.TurnRight.start -> UturnRight.TurnRight.turning [order 2] : [currentHeading == ROB_NORTH]
          | /headingRequest = ROB_EAST;
      UturnRight.TurnRight.start -> UturnRight.TurnRight.turning [order 4] : [currentHeading == ROB_SOUTH]
          | /headingRequest = ROB_WEST;
      UturnRight.TurnRight.turning -> UturnRight.TurnRight.finish : [(currentHeading...
          |  == headingRequest)...
          | && (targetReached == true)]
      UturnRight.TurnRight.start -> UturnRight.TurnRight.turning [order 3] : [currentHeading == ROB_WEST]
          | /headingRequest = ROB_NORTH;
      UturnRight.TurnRight.start -> UturnRight.TurnRight.turning [order 1] : [currentHeading == ROB_EAST]
          | /headingRequest = ROB_SOUTH;
    state forwardStep
      entry:
      //counter = 0;
      turnRequest = FORWARD;
      currentMove = FORWARD;
      du:
      //counter++;
    (default) -> UturnRight.TurnRight
    UturnRight.TurnRight -> UturnRight.finish [order 2] : [uTurnCounter == CONST_UTURN_CNT_THD]
    UturnRight.TurnRight -> UturnRight.forwardStep [order 1] : [hasChanged(uTurnCounter) ...
        | && (uTurnCounter == 1)]
    UturnRight.forwardStep -> UturnRight.TurnRight [order 2] : stopEvent
        | /currentMove = MOVE_U_TURN_RIGHT;
    UturnRight.forwardStep -> UturnRight.TurnRight [order 1] : [(hasChanged(completeStep))...
        | && (completeStep == true)]
        | /currentMove = MOVE_U_TURN_RIGHT;
  (default) -> init
  init -> Stop : [stableCounter >= CONST_MOVE_STABLE_CNT]
      | /headingRequest = ROB_NORTH;
  Stop -> (junction 9) : [hasChanged(moveRequest) ...
      | || (turnActive == false)]
  (junction 9) -> Stop [order 6] : [moveRequest == STOP]
      | /turnRequest = STOP;
      | currentMove = STOP;
  forward -> (junction 9) : [hasChanged(moveRequest)]
  (junction 9) -> TurnLeft [order 8] : [(moveRequest == MOVE_TURN_LEFT)]
      | /currentMove = MOVE_TURN_LEFT;
  (junction 9) -> forward [order 1] : [moveRequest == FORWARD]
      | /turnRequest = FORWARD;
      | currentMove = FORWARD;
  TurnLeft -> (junction 9) : [hasChanged(moveRequest) ...
      | || (turnActive == false)]
  (junction 9) -> backward [order 2] : [moveRequest == BACKWARD]
      | /turnRequest = BACKWARD;
      | currentMove = BACKWARD;
  (junction 9) -> UturnLeft [order 5] : [(moveRequest == MOVE_U_TURN_LEFT)]
      | /currentMove = MOVE_U_TURN_LEFT;
  backward -> (junction 9) : [hasChanged(moveRequest) ...
      | || (turnActive == false)]
  Uturn -> (junction 9) : [hasChanged(moveRequest) ...
      | || (turnActive == false)]
  UturnLeft -> (junction 9) : //[hasChanged(moveRequest) ...||
      | [(turnActive == false)]
  (junction 9) -> TurnRight [order 7] : [(moveRequest == MOVE_TURN_RIGHT)]
      | /currentMove = MOVE_TURN_RIGHT;
  (junction 9) -> Uturn [order 4] : [moveRequest == MOVE_U_TURN]
      | /currentMove = MOVE_U_TURN;
  UturnRight -> (junction 9) : //[hasChanged(moveRequest) ...||
      | [(turnActive == false)]
  TurnRight -> (junction 9) : [hasChanged(moveRequest) ...
      | || (turnActive == false)]
  (junction 9) -> UturnRight [order 3] : [(moveRequest == MOVE_U_TURN_RIGHT)]
      | /currentMove = MOVE_U_TURN_RIGHT;
  data: moveRequest input; currentHeading input; FORWARD input; BACKWARD input; STOP input; MOVE_TURN_LEFT input; MOVE_TURN_RIGHT input; MOVE_U_TURN_LEFT input; MOVE_U_TURN_RIGHT input; MOVE_U_TURN input; turnRequest output uint8; headingRequest output uint16; CCW input; CW input; ROB_NORTH input; ROB_SOUTH input; ROB_WEST input; ROB_EAST input; rawTheta input; turnActive local boolean; completeStep input; uTurnCounter local uint8; targetReached input; stableCounter local uint8; ROB_NONE input; currentMove local uint8; CAL_thetaGain constant uint8 =CAL_thetaGain; CAL_forwardThetaThd constant uint8 =CAL_forwardThetaThd; CONST_MOVE_STABLE_CNT constant uint8 =CONST_MOVE_STABLE_CNT; CONST_UTURN_CNT_THD constant uint8 =CONST_UTURN_CNT_THD
  events: refreshEvent input EITHER_EDGE_EVENT; stopEvent input EITHER_EDGE_EVENT
